simulink model "test_loopback_buf"  (Simulink 6.2)
settings: Solver=ode45  StartTime=0.0  StopTime=4000  RelTol=1e-3
undefined symbols (not defined in the file): Down, Up
libraries: xbsIndex_r3 x1383, xps_library x52, casper_library x37
(part 3 of 8)

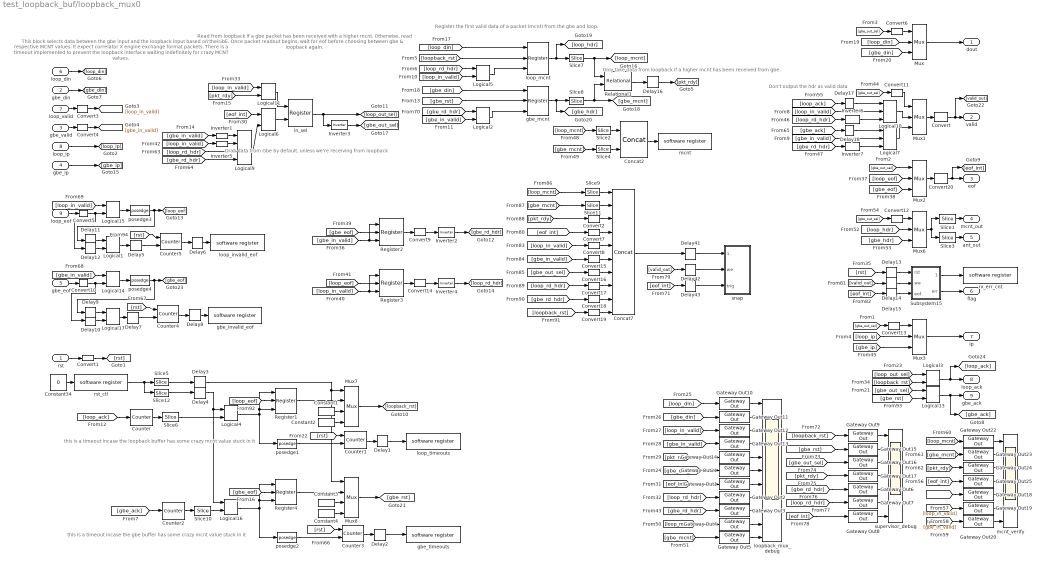
== system test_loopback_buf/loopback_mux0 ==
  note: Read from loopback if a gbe packet
      | has been received with a higher mcnt.
      | Otherwise, read from GbE.
      | Once packet readout begins, wait for eof
      | before choosing between gbe & loopback again.
  note: Only take data from loopback
      | if a higher mcnt has been
      | received from gbe.
  note: This block selects data between the gbe input
      | and the loopback input based on their respective MCNT values.
      | It expect correlator X engine exchange format packets.
      |
      | There is a timeout implemented to prevent the loopback interface
      | waiting indefinitely for crazy MCNT values.
  note: Don't output the hdr
      | as valid data
  note: this is a timeout incase
      | the gbe buffer has
      | some crazy mcnt value stuck in it
  note: this is a timeout incase
      | the loopback buffer has
      | some crazy mcnt value stuck in it
  note: Grab data from
      | Gbe by default,
      | unless we're receiving
      | from loopback
  note: Register the first valid
      | data of a packet (mcnt)
      | from the gbe and loop.
  rst : Inport  Port=1  LatchInput=off
  gbe_din : Inport  Port=2  LatchInput=off
  gbe_valid : Inport  Port=3  LatchInput=off
  gbe_ip : Inport  Port=4  LatchInput=off
  gbe_eof : Inport  Port=5  LatchInput=off
  loop_din : Inport  Port=6  LatchInput=off
  loop_valid : Inport  Port=7  LatchInput=off
  loop_ip : Inport  Port=8  LatchInput=off
  loop_eof : Inport  Port=9  LatchInput=off
  Concat2 : xbsIndex_r3/Concat  num_inputs=2  explicit_period=off  period=1  dbl_ovrd=off
  Concat7 : xbsIndex_r3/Concat  num_inputs=10  explicit_period=off  period=1  dbl_ovrd=off
  Constant1 : xbsIndex_r3/Constant  const=0  equ=P=C  arith_type=Boolean  n_bits=1  bin_pt=0  opselect=C  inp2=PCIN>>17  opr=+  inp1=P  carry=CIN  iostate=0  explicit_period=on  period=1  dbl_ovrd=off
  Constant2 : xbsIndex_r3/Constant  const=1  equ=P=C  arith_type=Boolean  n_bits=1  bin_pt=0  opselect=C  inp2=PCIN>>17  opr=+  inp1=P  carry=CIN  iostate=0  explicit_period=on  period=1  dbl_ovrd=off
  Constant3 : xbsIndex_r3/Constant  const=0  equ=P=C  arith_type=Boolean  n_bits=1  bin_pt=0  opselect=C  inp2=PCIN>>17  opr=+  inp1=P  carry=CIN  iostate=0  explicit_period=on  period=1  dbl_ovrd=off
  Constant34 : Constant  Value=0
  Constant4 : xbsIndex_r3/Constant  const=1  equ=P=C  arith_type=Boolean  n_bits=1  bin_pt=0  opselect=C  inp2=PCIN>>17  opr=+  inp1=P  carry=CIN  iostate=0  explicit_period=on  period=1  dbl_ovrd=off
  Convert{,1,9,14,20} (5 alike) : xbsIndex_r3/Convert  arith_type=Boolean  n_bits=8  bin_pt=6  quantization=Truncate  overflow=Wrap  latency=0  explicit_period=off  period=1  dbl_ovrd=off  show_param=off  inserted_by_tool=off  pipeline=off
      settings: xl_area=[0, 0, 0, 0, 0, 0, 0]
  Convert{3..5,10} (4 alike) : xbsIndex_r3/Convert  arith_type=Boolean  n_bits=1  bin_pt=0  quantization=Truncate  overflow=Wrap  latency=0  explicit_period=on  period=1  dbl_ovrd=off  show_param=off  inserted_by_tool=off  pipeline=off
      settings: xl_area=[0, 0, 0, 0, 0, 0, 0]
  Convert{2,6..8,11..13,15..19} (12 alike) : xbsIndex_r3/Convert  arith_type=Unsigned  n_bits=1  bin_pt=0  quantization=Truncate  overflow=Wrap  latency=0  explicit_period=off  period=1  dbl_ovrd=off  show_param=off  inserted_by_tool=off  pipeline=off
      settings: xl_area=[0, 0, 0, 0, 0, 0, 0]
  Counter : xbsIndex_r3/Counter  cnt_type=Free Running  n_bits=timeout_bits+1  bin_pt=0  arith_type=Unsigned  start_count=0  cnt_to=Inf  cnt_by_val=1  operation=Up  explicit_period=off  period=1  load_pin=off  rst=on  en=off  dbl_ovrd=off  show_param=off  use_rpm=on  gen_core=off
      settings: xl_area=[0, 0, 0, 0, 0, 0, 0]
  Counter{1,3..5} (4 alike) : xbsIndex_r3/Counter  cnt_type=Free Running  n_bits=27  bin_pt=0  arith_type=Unsigned  start_count=0  cnt_to=Inf  cnt_by_val=1  operation=Up  explicit_period=off  period=1  load_pin=off  rst=on  en=on  dbl_ovrd=off  show_param=off  use_rpm=on  gen_core=off
      settings: xl_area=[0, 0, 0, 0, 0, 0, 0]
  Counter2 : xbsIndex_r3/Counter  cnt_type=Free Running  n_bits=timeout_bits+1  bin_pt=0  arith_type=Unsigned  start_count=0  cnt_to=Inf  cnt_by_val=1  operation=Up  explicit_period=off  period=1  load_pin=off  rst=on  en=off  dbl_ovrd=off  show_param=off  use_rpm=on  gen_core=off
      settings: xl_area=[0, 0, 0, 0, 0, 0, 0]
  Delay{1..15} (15 alike) : xbsIndex_r3/Delay  latency=2  reg_retiming=on  explicit_period=on  period=1  en=off  accept_only_valid=off  init_zero=on  dbl_ovrd=off  show_param=off
      settings: xl_area=[0, 0, 0, 0, 0, 0, 0]
  Delay16 : xbsIndex_r3/Delay  latency=1  reg_retiming=on  explicit_period=on  period=1  en=off  accept_only_valid=off  init_zero=on  dbl_ovrd=off  show_param=off
      settings: xl_area=[0, 0, 0, 0, 0, 0, 0]
  Delay17 : xbsIndex_r3/Delay  latency=1  reg_retiming=on  explicit_period=on  period=1  en=off  accept_only_valid=off  init_zero=on  dbl_ovrd=off  show_param=off
      settings: xl_area=[0, 0, 0, 0, 0, 0, 0]
  Delay18 : xbsIndex_r3/Delay  latency=1  reg_retiming=on  explicit_period=on  period=1  en=off  accept_only_valid=off  init_zero=on  dbl_ovrd=off  show_param=off
      settings: xl_area=[0, 0, 0, 0, 0, 0, 0]
  Delay41 : xbsIndex_r3/Delay  latency=3  reg_retiming=on  explicit_period=on  period=1  en=off  accept_only_valid=off  init_zero=on  dbl_ovrd=off  show_param=off
      settings: xl_area=[0, 0, 0, 0, 0, 0, 0]
  Delay42 : xbsIndex_r3/Delay  latency=3  reg_retiming=on  explicit_period=on  period=1  en=off  accept_only_valid=off  init_zero=on  dbl_ovrd=off  show_param=off
      settings: xl_area=[0, 0, 0, 0, 0, 0, 0]
  Delay43 : xbsIndex_r3/Delay  latency=3  reg_retiming=on  explicit_period=on  period=1  en=off  accept_only_valid=off  init_zero=on  dbl_ovrd=off  show_param=off
      settings: xl_area=[0, 0, 0, 0, 0, 0, 0]
  Gateway Out{1..25} (25 alike) : xbsIndex_r3/Gateway Out  output_type=Double  nbits=8  bin_pt=6  arith_type=Boolean  quantization=Truncate  overflow=Wrap  hdl_port=on  timing_constraint=None  locs_specified=off  LOCs={}  needs_fixed_name=off  show_param=off
      settings: xl_area=[0, 0, 0, 0, 0, 0, 0]
  Inverter{1..7} (7 alike) : xbsIndex_r3/Inverter  latency=0  explicit_period=off  period=1  en=off  dbl_ovrd=off  show_param=off
      settings: xl_area=[0, 0, 0, 0, 0, 0, 0]
  Logical1 : xbsIndex_r3/Logical  logical_function=XOR  inputs=2  precision=Full  arith_type=Unsigned  n_bits=8  bin_pt=2  align_bp=on  latency=0  explicit_period=on  period=1  en=off  dbl_ovrd=off  show_param=off
      settings: xl_area=[0, 0, 0, 0, 0, 0, 0]
  Logical10 : xbsIndex_r3/Logical  logical_function=AND  inputs=3  precision=Full  arith_type=Unsigned  n_bits=8  bin_pt=2  align_bp=on  latency=0  explicit_period=on  period=1  en=off  dbl_ovrd=off  show_param=off
      settings: xl_area=[0, 0, 0, 0, 0, 0, 0]
  Logical11 : xbsIndex_r3/Logical  logical_function=AND  inputs=2  precision=Full  arith_type=Unsigned  n_bits=8  bin_pt=2  align_bp=on  latency=0  explicit_period=off  period=1  en=off  dbl_ovrd=off  show_param=off
      settings: xl_area=[0, 0, 0, 0, 0, 0, 0]
  Logical13 : xbsIndex_r3/Logical  logical_function=OR  inputs=2  precision=Full  arith_type=Unsigned  n_bits=8  bin_pt=2  align_bp=on  latency=0  explicit_period=off  period=1  en=off  dbl_ovrd=off  show_param=off
      settings: xl_area=[0, 0, 0, 0, 0, 0, 0]
  Logical14 : xbsIndex_r3/Logical  logical_function=AND  inputs=2  precision=Full  arith_type=Unsigned  n_bits=8  bin_pt=2  align_bp=on  latency=0  explicit_period=on  period=1  en=off  dbl_ovrd=off  show_param=off
      settings: xl_area=[0, 0, 0, 0, 0, 0, 0]
  Logical15 : xbsIndex_r3/Logical  logical_function=AND  inputs=2  precision=Full  arith_type=Unsigned  n_bits=8  bin_pt=2  align_bp=on  latency=0  explicit_period=on  period=1  en=off  dbl_ovrd=off  show_param=off
      settings: xl_area=[0, 0, 0, 0, 0, 0, 0]
  Logical16 : xbsIndex_r3/Logical  logical_function=OR  inputs=2  precision=Full  arith_type=Unsigned  n_bits=8  bin_pt=2  align_bp=on  latency=0  explicit_period=on  period=1  en=off  dbl_ovrd=off  show_param=off
      settings: xl_area=[0, 0, 0, 0, 0, 0, 0]
  Logical17 : xbsIndex_r3/Logical  logical_function=XOR  inputs=2  precision=Full  arith_type=Unsigned  n_bits=8  bin_pt=2  align_bp=on  latency=0  explicit_period=on  period=1  en=off  dbl_ovrd=off  show_param=off
      settings: xl_area=[0, 0, 0, 0, 0, 0, 0]
  Logical2 : xbsIndex_r3/Logical  logical_function=AND  inputs=2  precision=Full  arith_type=Unsigned  n_bits=8  bin_pt=2  align_bp=on  latency=0  explicit_period=off  period=1  en=off  dbl_ovrd=off  show_param=off
      settings: xl_area=[0, 0, 0, 0, 0, 0, 0]
  Logical3 : xbsIndex_r3/Logical  logical_function=OR  inputs=2  precision=Full  arith_type=Unsigned  n_bits=8  bin_pt=2  align_bp=on  latency=0  explicit_period=off  period=1  en=off  dbl_ovrd=off  show_param=off
      settings: xl_area=[0, 0, 0, 0, 0, 0, 0]
  Logical4 : xbsIndex_r3/Logical  logical_function=OR  inputs=2  precision=Full  arith_type=Unsigned  n_bits=8  bin_pt=2  align_bp=on  latency=0  explicit_period=on  period=1  en=off  dbl_ovrd=off  show_param=off
      settings: xl_area=[0, 0, 0, 0, 0, 0, 0]
  Logical5 : xbsIndex_r3/Logical  logical_function=AND  inputs=2  precision=Full  arith_type=Unsigned  n_bits=8  bin_pt=2  align_bp=on  latency=0  explicit_period=off  period=1  en=off  dbl_ovrd=off  show_param=off
      settings: xl_area=[0, 0, 0, 0, 0, 0, 0]
  Logical6 : xbsIndex_r3/Logical  logical_function=OR  inputs=2  precision=Full  arith_type=Unsigned  n_bits=8  bin_pt=2  align_bp=on  latency=0  explicit_period=off  period=1  en=off  dbl_ovrd=off  show_param=off
      settings: xl_area=[0, 0, 0, 0, 0, 0, 0]
  Logical7 : xbsIndex_r3/Logical  logical_function=AND  inputs=3  precision=Full  arith_type=Unsigned  n_bits=8  bin_pt=2  align_bp=on  latency=0  explicit_period=on  period=1  en=off  dbl_ovrd=off  show_param=off
      settings: xl_area=[0, 0, 0, 0, 0, 0, 0]
  Logical9 : xbsIndex_r3/Logical  logical_function=AND  inputs=4  precision=Full  arith_type=Unsigned  n_bits=8  bin_pt=2  align_bp=on  latency=0  explicit_period=on  period=1  en=off  dbl_ovrd=off  show_param=off
      settings: xl_area=[0, 0, 0, 0, 0, 0, 0]
  Mux{,1,3,6} (4 alike) : xbsIndex_r3/Mux  inputs=2  precision=Full  arith_type="Signed  (2's comp)"  n_bits=8  bin_pt=2  quantization=Truncate  overflow=Wrap  latency=0  explicit_period=off  period=1  en=off  dbl_ovrd=off  show_param=off  mux_type=off  use_rpm=off  gen_core=off
      settings: xl_area=[0, 0, 0, 0, 0, 0, 0]
  Mux2 : xbsIndex_r3/Mux  inputs=2  precision=Full  arith_type="Signed  (2's comp)"  n_bits=8  bin_pt=2  quantization=Truncate  overflow=Wrap  latency=0  explicit_period=on  period=1  en=off  dbl_ovrd=off  show_param=off  mux_type=off  use_rpm=off  gen_core=off
      settings: xl_area=[0, 0, 0, 0, 0, 0, 0]
  Mux7 : xbsIndex_r3/Mux  inputs=3  precision=Full  arith_type="Signed  (2's comp)"  n_bits=8  bin_pt=2  quantization=Truncate  overflow=Wrap  latency=2  explicit_period=off  period=1  en=off  dbl_ovrd=off  show_param=off  mux_type=off  use_rpm=off  gen_core=off
      settings: xl_area=[0, 0, 0, 0, 0, 0, 0]
  Mux8 : xbsIndex_r3/Mux  inputs=3  precision=Full  arith_type="Signed  (2's comp)"  n_bits=8  bin_pt=2  quantization=Truncate  overflow=Wrap  latency=2  explicit_period=off  period=1  en=off  dbl_ovrd=off  show_param=off  mux_type=off  use_rpm=off  gen_core=off
      settings: xl_area=[0, 0, 0, 0, 0, 0, 0]
  Register{1..4} (4 alike) : xbsIndex_r3/Register  init=0  reg_only_valid=off  explicit_period=on  period=1  rst=on  en=on  out_en=off  dbl_ovrd=off  show_param=off
      settings: xl_area=[0, 0, 0, 0, 0, 0, 0]
  Relational1 : xbsIndex_r3/Relational  mode=a<b  latency=1  explicit_period=off  period=1  en=off  dbl_ovrd=off  show_param=off
      settings: xl_area=[0, 0, 0, 0, 0, 0, 0]
  Slice1 : xbsIndex_r3/Slice  mode=Lower Bit Location + Width  nbits=48  bit1=0  base1=MSB of Input  bit0=16  base0=LSB of Input  boolean_output=off  explicit_period=off  period=1  dbl_ovrd=off
  Slice10 : xbsIndex_r3/Slice  mode=Upper Bit Location + Width  nbits=1  bit1=0  base1=MSB of Input  bit0=1  base0=LSB of Input  boolean_output=on  explicit_period=off  period=1  dbl_ovrd=off
  Slice11 : xbsIndex_r3/Slice  mode=Lower Bit Location + Width  nbits=12  bit1=0  base1=MSB of Input  bit0=0  base0=LSB of Input  boolean_output=off  explicit_period=off  period=1  dbl_ovrd=off
  Slice12 : xbsIndex_r3/Slice  mode=Lower Bit Location + Width  nbits=1  bit1=0  base1=MSB of Input  bit0=0  base0=LSB of Input  boolean_output=on  explicit_period=off  period=1  dbl_ovrd=off
  Slice2 : xbsIndex_r3/Slice  mode=Lower Bit Location + Width  nbits=16  bit1=0  base1=MSB of Input  bit0=0  base0=LSB of Input  boolean_output=off  explicit_period=off  period=1  dbl_ovrd=off
  Slice3 : xbsIndex_r3/Slice  mode=Lower Bit Location + Width  nbits=16  bit1=0  base1=MSB of Input  bit0=0  base0=LSB of Input  boolean_output=off  explicit_period=off  period=1  dbl_ovrd=off
  Slice4 : xbsIndex_r3/Slice  mode=Lower Bit Location + Width  nbits=16  bit1=0  base1=MSB of Input  bit0=0  base0=LSB of Input  boolean_output=off  explicit_period=off  period=1  dbl_ovrd=off
  Slice5 : xbsIndex_r3/Slice  mode=Lower Bit Location + Width  nbits=2  bit1=0  base1=MSB of Input  bit0=1  base0=LSB of Input  boolean_output=off  explicit_period=off  period=1  dbl_ovrd=off
  Slice6 : xbsIndex_r3/Slice  mode=Upper Bit Location + Width  nbits=1  bit1=0  base1=MSB of Input  bit0=1  base0=LSB of Input  boolean_output=on  explicit_period=off  period=1  dbl_ovrd=off
  Slice7 : xbsIndex_r3/Slice  mode=Upper Bit Location + Width  nbits=48  bit1=0  base1=MSB of Input  bit0=0  base0=LSB of Input  boolean_output=off  explicit_period=off  period=1  dbl_ovrd=off
  Slice8 : xbsIndex_r3/Slice  mode=Upper Bit Location + Width  nbits=48  bit1=0  base1=MSB of Input  bit0=0  base0=LSB of Input  boolean_output=off  explicit_period=off  period=1  dbl_ovrd=off
  Slice9 : xbsIndex_r3/Slice  mode=Lower Bit Location + Width  nbits=12  bit1=0  base1=MSB of Input  bit0=0  base0=LSB of Input  boolean_output=off  explicit_period=off  period=1  dbl_ovrd=off
  Subsystem15 : Subsystem  mask{payload_len=payload_len}
      mask init:
      | fmtstr = sprintf('Payload Length: %d', payload_len);
      | set_param(gcb, 'AttributesFormatString', fmtstr);
      settings: AttributesFormatString=Payload Length: 32
  gbe_invalid_eof : xps_library/software register  Tag=xps:sw_reg  io_dir=To Processor  arith_type=Unsigned  bitwidth=32  bin_pt=0  sample_period=1  gw_name=b_2x_8a_r310_a_loopback_mux0_gbe_invalid_eof_user_data_in
  gbe_mcnt : xbsIndex_r3/Register  init=0  reg_only_valid=off  explicit_period=on  period=1  rst=on  en=on  out_en=off  dbl_ovrd=off  show_param=off
      settings: xl_area=[0, 0, 0, 0, 0, 0, 0]
  gbe_timeouts : xps_library/software register  Tag=xps:sw_reg  io_dir=To Processor  arith_type=Unsigned  bitwidth=32  bin_pt=0  sample_period=1  gw_name=b_2x_8a_r310_a_loopback_mux0_gbe_timeouts_user_data_in
  in_sel : xbsIndex_r3/Register  init=0  reg_only_valid=off  explicit_period=on  period=1  rst=off  en=on  out_en=off  dbl_ovrd=off  show_param=off
      settings: xl_area=[0, 0, 0, 0, 0, 0, 0]
  loop_invalid_eof : xps_library/software register  Tag=xps:sw_reg  io_dir=To Processor  arith_type=Unsigned  bitwidth=32  bin_pt=0  sample_period=1  gw_name=b_2x_8a_r310_a_loopback_mux0_loop_invalid_eof_user_data_in
  loop_mcnt : xbsIndex_r3/Register  init=0  reg_only_valid=off  explicit_period=on  period=1  rst=on  en=on  out_en=off  dbl_ovrd=off  show_param=off
      settings: xl_area=[0, 0, 0, 0, 0, 0, 0]
  loop_timeouts : xps_library/software register  Tag=xps:sw_reg  io_dir=To Processor  arith_type=Unsigned  bitwidth=32  bin_pt=0  sample_period=1  gw_name=b_2x_8a_r310_a_loopback_mux0_loop_timeouts_user_data_in
  loopback_mux_debug : Scope  NumInputPorts=11
      settings: YMin=300~190.95~0~0.95~0.95~-1~-1~-1~-5~-5~-5  YMax=525~211.05~1~1.05~1.05~1~1~1~5~5~5  SaveName=ScopeData7
  mcnt : xps_library/software register  Tag=xps:sw_reg  io_dir=To Processor  arith_type=Unsigned  bitwidth=32  bin_pt=0  sample_period=1  gw_name=b_2x_8a_r310_a_loopback_mux0_mcnt_user_data_in
  mcnt_verify : Scope  NumInputPorts=7
      settings: YMin=300~190.95~0~-5~-5~-5~-5  YMax=525~211.05~1~5~5~5~5  SaveName=ScopeData2
  posedge{1..4} (4 alike) : casper_library/Misc/posedge  Tag=Rising Edge Detector
  rst_ctl : xps_library/software register  Tag=xps:sw_reg  io_dir=From Processor  arith_type=Unsigned  bitwidth=32  bin_pt=0  sample_period=1  gw_name=b_2x_8a_r310_a_loopback_mux0_rst_ctl_user_data_out
  rx_err_cnt : xps_library/software register  Tag=xps:sw_reg  io_dir=To Processor  arith_type=Unsigned  bitwidth=32  bin_pt=0  sample_period=1  gw_name=b_2x_8a_r310_a_loopback_mux0_rx_err_cnt_user_data_in
  snap : Subsystem  mask{nsamples=12}
      mask prompts: nsamples "Number of Samples (2^?)"
  supervisor_debug : Scope  NumInputPorts=7
      settings: YMin=300~190.95~0~-5~-5~-5~-5  YMax=525~211.05~1~5~5~5~5  SaveName=ScopeData18
  dout : Outport
  valid : Outport  Port=2
  eof : Outport  Port=3
  mcnt_out : Outport  Port=4
  ant_out : Outport  Port=5
  flag : Outport  Port=6
  ip : Outport  Port=7
  loop_ack : Outport  Port=8
  gbe_ack : Outport  Port=9
  wires:
  Mux/1 -> dout/1
  Mux1/1 -> Convert/1
  Mux2/1 -> Convert20/1
  gbe_valid/1 -> Convert4/1
  loop_valid/1 -> Convert3/1
  Convert/1 -> valid/1, [valid_out]
  Slice2/1 -> Concat2/1
  Slice4/1 -> Concat2/2
  Concat2/1 -> mcnt/1
  Convert6/1 -> Mux/1
  [gbe_out_sel] -> Convert6/1
  [gbe_out_sel] -> Mux2/1
  Gateway Out12/1 -> loopback_mux_debug/3
  Gateway Out13/1 -> loopback_mux_debug/4
  Gateway Out14/1 -> loopback_mux_debug/5
  Gateway Out21/1 -> loopback_mux_debug/6
  Convert3/1 -> [loop_in_valid]
  Convert4/1 -> [gbe_in_valid]
  Relational1/1 -> Delay16/1
  loop_din/1 -> [loop_din]
  gbe_din/1 -> [gbe_din]
  [loop_din] -> Mux/2
  [gbe_din] -> Mux/3
  [gbe_din] -> Gateway Out11/1
  [loop_din] -> Gateway Out10/1
  [loop_in_valid] -> Gateway Out12/1
  [gbe_in_valid] -> Gateway Out13/1
  [gbe_out_sel] -> Gateway Out21/1
  [pkt_rdy] -> Gateway Out14/1
  Gateway Out1/1 -> loopback_mux_debug/7
  [eof_int] -> Gateway Out1/1
  [loop_rd_hdr] -> Gateway Out2/1
  Gateway Out2/1 -> loopback_mux_debug/8
  [loop_eof] -> Mux2/2
  loop_eof/1 -> Convert5/1
  gbe_eof/1 -> Convert10/1
  [gbe_eof] -> Mux2/3
  Gateway Out3/1 -> loopback_mux_debug/9
  [gbe_rd_hdr] -> Gateway Out3/1
  [gbe_out_sel] -> Convert11/1
  Convert11/1 -> Mux1/1
  loop_ip/1 -> [loop_ip]
  gbe_ip/1 -> [gbe_ip]
  Mux3/1 -> ip/1
  [loop_ip] -> Mux3/2
  [gbe_ip] -> Mux3/3
  [gbe_out_sel] -> Convert13/1
  Convert13/1 -> Mux3/1
  [loop_mcnt] -> Slice2/1
  [gbe_mcnt] -> Slice4/1
  Gateway Out10/1 -> loopback_mux_debug/1
  Gateway Out11/1 -> loopback_mux_debug/2
  Gateway Out4/1 -> loopback_mux_debug/10
  Gateway Out5/1 -> loopback_mux_debug/11
  [loop_mcnt] -> Gateway Out4/1
  [gbe_mcnt] -> Gateway Out5/1
  Gateway Out24/1 -> mcnt_verify/3
  Gateway Out22/1 -> mcnt_verify/1
  Gateway Out23/1 -> mcnt_verify/2
  Gateway Out25/1 -> mcnt_verify/4
  Gateway Out18/1 -> mcnt_verify/5
  Gateway Out19/1 -> mcnt_verify/6
  Gateway Out20/1 -> mcnt_verify/7
  [gbe_out_sel] -> Gateway Out20/1
  [gbe_in_valid] -> Gateway Out19/1
  [loop_in_valid] -> Gateway Out18/1
  [eof_int] -> Gateway Out25/1
  [loop_mcnt] -> Gateway Out22/1
  [gbe_mcnt] -> Gateway Out23/1
  [pkt_rdy] -> Gateway Out24/1
  Slice7/1 -> Relational1/1, [loop_mcnt]
  Slice8/1 -> Relational1/2, [gbe_mcnt]
  Slice1/1 -> mcnt_out/1
  Slice3/1 -> ant_out/1
  Convert12/1 -> Mux6/1
  [gbe_out_sel] -> Convert12/1
  [loop_hdr] -> Mux6/2
  [gbe_hdr] -> Mux6/3
  Mux6/1 -> Slice1/1, Slice3/1
  [loop_in_valid] -> Logical10/2
  [loop_ack] -> Delay17/1
  [gbe_ack] -> Delay18/1
  [gbe_in_valid] -> Logical7/2
  Logical7/1 -> Mux1/3
  Counter2/1 -> Slice10/1
  [gbe_ack] -> Counter2/1
  [rst] -> Counter3/1
  Counter3/1 -> Delay2/1
  Logical16/1 -> Register4/1, Register4/3, posedge2/1
  Logical14/1 -> posedge4/1
  Logical15/1 -> posedge3/1
  Convert5/1 -> Logical15/2, Delay12/1
  Convert10/1 -> Logical14/2, Delay10/1
  [gbe_in_valid] -> Logical14/1
  [loop_in_valid] -> Logical15/1
  Slice10/1 -> Logical16/2
  Gateway Out16/1 -> supervisor_debug/3
  Gateway Out9/1 -> supervisor_debug/1
  Gateway Out15/1 -> supervisor_debug/2
  Gateway Out17/1 -> supervisor_debug/4
  Gateway Out6/1 -> supervisor_debug/5
  Gateway Out7/1 -> supervisor_debug/6
  Gateway Out8/1 -> supervisor_debug/7
  [loopback_rst] -> Gateway Out9/1
  [gbe_rst] -> Gateway Out15/1
  [gbe_out_sel] -> Gateway Out16/1
  [pkt_rdy] -> Gateway Out17/1
  [gbe_rd_hdr] -> Gateway Out6/1
  [loop_rd_hdr] -> Gateway Out7/1
  [eof_int] -> Gateway Out8/1
  Logical3/1 -> loop_ack/1, [loop_ack]
  Logical13/1 -> gbe_ack/1, [gbe_ack]
  rst/1 -> Convert1/1
  Subsystem15/1(err_cnt) -> rx_err_cnt/1
  Subsystem15/2(err) -> flag/1
  [rst] -> Delay13/1
  [valid_out] -> Delay14/1
  [eof_int] -> Delay15/1
  Counter/1 -> Slice6/1
  Slice6/1 -> Logical4/2
  [loop_ack] -> Counter/1
  [rst] -> Counter1/1
  Counter1/1 -> Delay1/1
  Logical4/1 -> Register1/1, Register1/3, posedge1/1
  [pkt_rdy] -> Logical11/2
  [eof_int] -> Logical6/1
  Inverter3/1 -> [gbe_out_sel]
  in_sel/1 -> Inverter3/1, [loop_out_sel]
  Logical6/1 -> in_sel/2
  [loop_in_valid] -> Logical11/1
  Register2/1 -> Convert9/1
  Convert9/1 -> Inverter2/1
  Inverter2/1 -> [gbe_rd_hdr]
  [gbe_eof] -> Register2/2
  Register3/1 -> Convert14/1
  Convert14/1 -> Inverter4/1
  Inverter4/1 -> [loop_rd_hdr]
  [loop_eof] -> Register3/2
  Logical11/1 -> in_sel/1
  [gbe_in_valid] -> Register2/1, Register2/3
  [loop_in_valid] -> Register3/1, Register3/3
  [gbe_in_valid] -> Inverter1/1
  [loop_in_valid] -> Inverter5/1
  Logical9/1 -> Logical6/2
  Inverter1/1 -> Logical9/1
  Inverter5/1 -> Logical9/2
  [loop_rd_hdr] -> Logical9/3
  [gbe_rd_hdr] -> Logical9/4
  gbe_mcnt/1 -> Slice8/1, [gbe_hdr]
  loop_mcnt/1 -> Slice7/1, [loop_hdr]
  Logical5/1 -> loop_mcnt/3
  [loop_rd_hdr] -> Logical5/1
  [gbe_rd_hdr] -> Logical2/1
  [loop_in_valid] -> Logical5/2
  [gbe_in_valid] -> Logical2/2
  [loop_din] -> loop_mcnt/1
  [gbe_din] -> gbe_mcnt/1
  Concat7/1 -> Delay41/1
  Delay42/1 -> snap/2(we)
  Delay43/1 -> snap/3(trig)
  Delay41/1 -> snap/1(data_in)
  [valid_out] -> Delay42/1
  [eof_int] -> Delay43/1
  [loop_mcnt] -> Slice9/1
  [gbe_mcnt] -> Slice11/1
  Slice9/1 -> Concat7/1
  Slice11/1 -> Concat7/2
  [pkt_rdy] -> Convert2/1
  [eof_int] -> Convert7/1
  [loop_in_valid] -> Convert8/1
  [gbe_in_valid] -> Convert15/1
  [gbe_out_sel] -> Convert16/1
  [loop_rd_hdr] -> Convert17/1
  [gbe_rd_hdr] -> Convert18/1
  [loopback_rst] -> Convert19/1
  [loop_eof] -> Register1/2
  [gbe_eof] -> Register4/2
  [loop_out_sel] -> Logical3/1
  [gbe_out_sel] -> Logical13/1
  [loopback_rst] -> Logical3/2
  [gbe_rst] -> Logical13/2
  Mux7/1 -> [loopback_rst]
  Register1/1 -> Mux7/2
  Mux8/1 -> [gbe_rst]
  Register4/1 -> Mux8/2
  Constant1/1 -> Mux7/3
  Constant34/1 -> rst_ctl/1
  rst_ctl/1 -> Slice5/1, Slice12/1
  Slice5/1 -> Delay3/1
  Convert1/1 -> [rst]
  Slice12/1 -> Delay4/1
  [loopback_rst] -> loop_mcnt/2
  [gbe_rst] -> gbe_mcnt/2
  Convert2/1 -> Concat7/3
  Convert7/1 -> Concat7/4
  Convert8/1 -> Concat7/5
  Convert15/1 -> Concat7/6
  Convert16/1 -> Concat7/7
  Convert17/1 -> Concat7/8
  Convert18/1 -> Concat7/9
  Convert19/1 -> Concat7/10
  Convert20/1 -> [eof_int], eof/1
  posedge1/1 -> Counter1/2
  posedge2/1 -> Counter3/2
  posedge3/1 -> [loop_eof], Delay11/1
  posedge4/1 -> [gbe_eof], Delay9/1
  [rst] -> Counter5/1
  Counter5/1 -> Delay6/1
  Logical1/1 -> Delay5/1
  Constant2/1 -> Mux7/4
  Constant3/1 -> Mux8/3
  Constant4/1 -> Mux8/4
  Delay1/1 -> loop_timeouts/1
  Delay2/1 -> gbe_timeouts/1
  Delay3/1 -> Mux7/1, Mux8/1
  Delay4/1 -> Logical4/1, Logical16/1
  Delay5/1 -> Counter5/2
  Delay6/1 -> loop_invalid_eof/1
  [rst] -> Counter4/1
  Counter4/1 -> Delay8/1
  Logical17/1 -> Delay7/1
  Delay7/1 -> Counter4/2
  Delay8/1 -> gbe_invalid_eof/1
  Delay9/1 -> Logical17/1
  Delay10/1 -> Logical17/2
  Delay11/1 -> Logical1/1
  Delay12/1 -> Logical1/2
  Delay13/1 -> Subsystem15/1(rst)
  Delay14/1 -> Subsystem15/2(we)
  Delay15/1 -> Subsystem15/3(eof)
  Logical2/1 -> gbe_mcnt/3
  Delay16/1 -> [pkt_rdy]
  Delay17/1 -> Logical10/1
  Delay18/1 -> Logical7/1
  Inverter6/1 -> Logical10/3
  [loop_rd_hdr] -> Inverter6/1
  [gbe_rd_hdr] -> Inverter7/1
  Inverter7/1 -> Logical7/3
  Logical10/1 -> Mux1/2

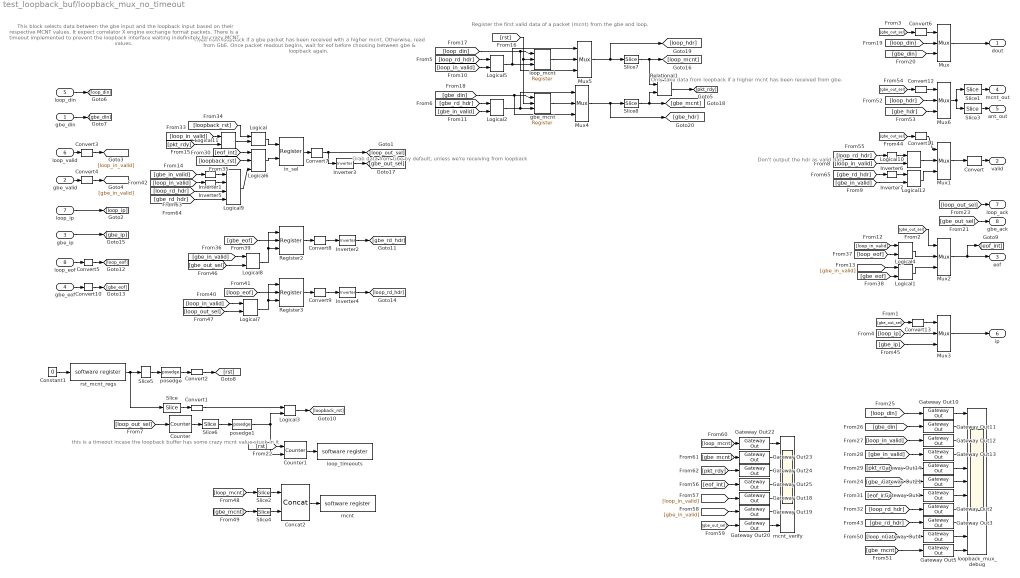
== system test_loopback_buf/loopback_mux_no_timeout ==
  note: Read from loopback if a gbe packet
      | has been received with a higher mcnt.
      | Otherwise, read from GbE.
      | Once packet readout begins, wait for eof
      | before choosing between gbe & loopback again.
  note: Register the first valid
      | data of a packet (mcnt)
      | from the gbe and loop.
  note: Only take data from loopback
      | if a higher mcnt has been
      | received from gbe.
  note: This block selects data between the gbe input
      | and the loopback input based on their respective MCNT values.
      | It expect correlator X engine exchange format packets.
      |
      | There is a timeout implemented to prevent the loopback interface
      | waiting indefinitely for crazy MCNT values.
  note: this is a timeout incase
      | the loopback buffer has
      | some crazy mcnt value stuck in it
  note: Grab data from
      | Gbe by default,
      | unless we're receiving
      | from loopback
  note: Don't output the hdr
      | as valid data
  gbe_din : Inport  Port=1  LatchInput=off
  gbe_valid : Inport  Port=2  LatchInput=off
  gbe_ip : Inport  Port=3  LatchInput=off
  gbe_eof : Inport  Port=4  LatchInput=off
  loop_din : Inport  Port=5  LatchInput=off
  loop_valid : Inport  Port=6  LatchInput=off
  loop_ip : Inport  Port=7  LatchInput=off
  loop_eof : Inport  Port=8  LatchInput=off
  Concat2 : xbsIndex_r3/Concat  num_inputs=2  explicit_period=off  period=1  dbl_ovrd=off
  Constant1 : Constant  Value=0
  Convert{,1..2,7..9} (6 alike) : xbsIndex_r3/Convert  arith_type=Boolean  n_bits=8  bin_pt=6  quantization=Truncate  overflow=Wrap  latency=0  explicit_period=off  period=1  dbl_ovrd=off  show_param=off  inserted_by_tool=off  pipeline=off
      settings: xl_area=[0, 0, 0, 0, 0, 0, 0]
  Convert{3..5,10} (4 alike) : xbsIndex_r3/Convert  arith_type=Boolean  n_bits=1  bin_pt=0  quantization=Truncate  overflow=Wrap  latency=0  explicit_period=on  period=1  dbl_ovrd=off  show_param=off  inserted_by_tool=off  pipeline=off
      settings: xl_area=[0, 0, 0, 0, 0, 0, 0]
  Convert{6,11..13} (4 alike) : xbsIndex_r3/Convert  arith_type=Unsigned  n_bits=1  bin_pt=0  quantization=Truncate  overflow=Wrap  latency=0  explicit_period=off  period=1  dbl_ovrd=off  show_param=off  inserted_by_tool=off  pipeline=off
      settings: xl_area=[0, 0, 0, 0, 0, 0, 0]
  Counter : xbsIndex_r3/Counter  cnt_type=Free Running  n_bits=loopback_timeout + 1  bin_pt=0  arith_type=Unsigned  start_count=0  cnt_to=Inf  cnt_by_val=1  operation=Up  explicit_period=off  period=1  load_pin=off  rst=on  en=off  dbl_ovrd=off  show_param=off  use_rpm=on  gen_core=off
      settings: xl_area=[0, 0, 0, 0, 0, 0, 0]
  Counter1 : xbsIndex_r3/Counter  cnt_type=Free Running  n_bits=27  bin_pt=0  arith_type=Unsigned  start_count=0  cnt_to=Inf  cnt_by_val=1  operation=Up  explicit_period=off  period=1  load_pin=off  rst=on  en=on  dbl_ovrd=off  show_param=off  use_rpm=on  gen_core=off
      settings: xl_area=[0, 0, 0, 0, 0, 0, 0]
  Gateway Out{1..5,10..14,18..25} (18 alike) : xbsIndex_r3/Gateway Out  output_type=Double  nbits=8  bin_pt=6  arith_type=Boolean  quantization=Truncate  overflow=Wrap  hdl_port=on  timing_constraint=None  locs_specified=off  LOCs={}  needs_fixed_name=off  show_param=off
      settings: xl_area=[0, 0, 0, 0, 0, 0, 0]
  Inverter{1..7} (7 alike) : xbsIndex_r3/Inverter  latency=0  explicit_period=off  period=1  en=off  dbl_ovrd=off  show_param=off
      settings: xl_area=[0, 0, 0, 0, 0, 0, 0]
  Logical : xbsIndex_r3/Logical  logical_function=OR  inputs=2  precision=Full  arith_type=Unsigned  n_bits=8  bin_pt=2  align_bp=on  latency=0  explicit_period=off  period=1  en=off  dbl_ovrd=off  show_param=off
      settings: xl_area=[0, 0, 0, 0, 0, 0, 0]
  Logical{1,4,7..8,10} (5 alike) : xbsIndex_r3/Logical  logical_function=AND  inputs=2  precision=Full  arith_type=Unsigned  n_bits=8  bin_pt=2  align_bp=on  latency=0  explicit_period=on  period=1  en=off  dbl_ovrd=off  show_param=off
      settings: xl_area=[0, 0, 0, 0, 0, 0, 0]
  Logical{2,5,11..12} (4 alike) : xbsIndex_r3/Logical  logical_function=AND  inputs=2  precision=Full  arith_type=Unsigned  n_bits=8  bin_pt=2  align_bp=on  latency=0  explicit_period=off  period=1  en=off  dbl_ovrd=off  show_param=off
      settings: xl_area=[0, 0, 0, 0, 0, 0, 0]
  Logical3 : xbsIndex_r3/Logical  logical_function=OR  inputs=2  precision=Full  arith_type=Unsigned  n_bits=8  bin_pt=2  align_bp=on  latency=0  explicit_period=off  period=1  en=off  dbl_ovrd=off  show_param=off
      settings: xl_area=[0, 0, 0, 0, 0, 0, 0]
  Logical6 : xbsIndex_r3/Logical  logical_function=OR  inputs=3  precision=Full  arith_type=Unsigned  n_bits=8  bin_pt=2  align_bp=on  latency=0  explicit_period=off  period=1  en=off  dbl_ovrd=off  show_param=off
      settings: xl_area=[0, 0, 0, 0, 0, 0, 0]
  Logical9 : xbsIndex_r3/Logical  logical_function=AND  inputs=4  precision=Full  arith_type=Unsigned  n_bits=8  bin_pt=2  align_bp=on  latency=0  explicit_period=on  period=1  en=off  dbl_ovrd=off  show_param=off
      settings: xl_area=[0, 0, 0, 0, 0, 0, 0]
  Mux{,1,3..6} (6 alike) : xbsIndex_r3/Mux  inputs=2  precision=Full  arith_type="Signed  (2's comp)"  n_bits=8  bin_pt=2  quantization=Truncate  overflow=Wrap  latency=0  explicit_period=off  period=1  en=off  dbl_ovrd=off  show_param=off  mux_type=off  use_rpm=off  gen_core=off
      settings: xl_area=[0, 0, 0, 0, 0, 0, 0]
  Mux2 : xbsIndex_r3/Mux  inputs=2  precision=Full  arith_type="Signed  (2's comp)"  n_bits=8  bin_pt=2  quantization=Truncate  overflow=Wrap  latency=0  explicit_period=on  period=1  en=off  dbl_ovrd=off  show_param=off  mux_type=off  use_rpm=off  gen_core=off
      settings: xl_area=[0, 0, 0, 0, 0, 0, 0]
  Register2 : xbsIndex_r3/Register  init=0  reg_only_valid=off  explicit_period=on  period=1  rst=on  en=on  out_en=off  dbl_ovrd=off  show_param=off
      settings: xl_area=[0, 0, 0, 0, 0, 0, 0]
  Register3 : xbsIndex_r3/Register  init=0  reg_only_valid=off  explicit_period=on  period=1  rst=on  en=on  out_en=off  dbl_ovrd=off  show_param=off
      settings: xl_area=[0, 0, 0, 0, 0, 0, 0]
  Relational1 : xbsIndex_r3/Relational  mode=a<b  latency=0  explicit_period=off  period=1  en=off  dbl_ovrd=off  show_param=off
      settings: xl_area=[0, 0, 0, 0, 0, 0, 0]
  Slice : xbsIndex_r3/Slice  mode=Lower Bit Location + Width  nbits=1  bit1=0  base1=MSB of Input  bit0=1  base0=LSB of Input  boolean_output=off  explicit_period=off  period=1  dbl_ovrd=off
  Slice1 : xbsIndex_r3/Slice  mode=Lower Bit Location + Width  nbits=48  bit1=0  base1=MSB of Input  bit0=16  base0=LSB of Input  boolean_output=off  explicit_period=off  period=1  dbl_ovrd=off
  Slice2 : xbsIndex_r3/Slice  mode=Lower Bit Location + Width  nbits=16  bit1=0  base1=MSB of Input  bit0=0  base0=LSB of Input  boolean_output=off  explicit_period=off  period=1  dbl_ovrd=off
  Slice3 : xbsIndex_r3/Slice  mode=Lower Bit Location + Width  nbits=16  bit1=0  base1=MSB of Input  bit0=0  base0=LSB of Input  boolean_output=off  explicit_period=off  period=1  dbl_ovrd=off
  Slice4 : xbsIndex_r3/Slice  mode=Lower Bit Location + Width  nbits=16  bit1=0  base1=MSB of Input  bit0=0  base0=LSB of Input  boolean_output=off  explicit_period=off  period=1  dbl_ovrd=off
  Slice5 : xbsIndex_r3/Slice  mode=Lower Bit Location + Width  nbits=1  bit1=0  base1=MSB of Input  bit0=0  base0=LSB of Input  boolean_output=off  explicit_period=off  period=1  dbl_ovrd=off
  Slice6 : xbsIndex_r3/Slice  mode=Upper Bit Location + Width  nbits=1  bit1=0  base1=MSB of Input  bit0=1  base0=LSB of Input  boolean_output=on  explicit_period=off  period=1  dbl_ovrd=off
  Slice7 : xbsIndex_r3/Slice  mode=Upper Bit Location + Width  nbits=48  bit1=0  base1=MSB of Input  bit0=0  base0=LSB of Input  boolean_output=off  explicit_period=off  period=1  dbl_ovrd=off
  Slice8 : xbsIndex_r3/Slice  mode=Upper Bit Location + Width  nbits=48  bit1=0  base1=MSB of Input  bit0=0  base0=LSB of Input  boolean_output=off  explicit_period=off  period=1  dbl_ovrd=off
  gbe_mcnt : xbsIndex_r3/Register  init=0  reg_only_valid=off  explicit_period=on  period=1  rst=on  en=on  out_en=off  dbl_ovrd=off  show_param=off
      settings: xl_area=[0, 0, 0, 0, 0, 0, 0]
  in_sel : xbsIndex_r3/Register  init=0  reg_only_valid=off  explicit_period=on  period=1  rst=off  en=on  out_en=off  dbl_ovrd=off  show_param=off
      settings: xl_area=[0, 0, 0, 0, 0, 0, 0]
  loop_mcnt : xbsIndex_r3/Register  init=0  reg_only_valid=off  explicit_period=on  period=1  rst=on  en=on  out_en=off  dbl_ovrd=off  show_param=off
      settings: xl_area=[0, 0, 0, 0, 0, 0, 0]
  loop_timeouts : xps_library/software register  Tag=xps:sw_reg  io_dir=To Processor  arith_type=Unsigned  bitwidth=32  bin_pt=0  sample_period=1  gw_name=test_loopback_buf_loopback_mux_no_timeout_loop_timeouts_user_data_in
  loopback_mux_debug : Scope  NumInputPorts=11
      settings: YMin=300~190.95~0~0.95~0.95~-1~-1~-1~-5~-5~-5  YMax=525~211.05~1~1.05~1.05~1~1~1~5~5~5  SaveName=ScopeData7
  mcnt : xps_library/software register  Tag=xps:sw_reg  io_dir=To Processor  arith_type=Unsigned  bitwidth=32  bin_pt=0  sample_period=1  gw_name=test_loopback_buf_loopback_mux_no_timeout_mcnt_user_data_in
  mcnt_verify : Scope  NumInputPorts=7
      settings: YMin=300~190.95~0~-5~-5~-5~-5  YMax=525~211.05~1~5~5~5~5  SaveName=ScopeData2
  posedge : casper_library/Misc/posedge  Tag=Rising Edge Detector
  posedge1 : casper_library/Misc/posedge  Tag=Rising Edge Detector
  rst_mcnt_regs : xps_library/software register  Tag=xps:sw_reg  io_dir=From Processor  arith_type=Unsigned  bitwidth=32  bin_pt=0  sample_period=1  gw_name=test_loopback_buf_loopback_mux_no_timeout_rst_mcnt_regs_user_data_out
  dout : Outport
  valid : Outport  Port=2
  eof : Outport  Port=3
  mcnt_out : Outport  Port=4
  ant_out : Outport  Port=5
  ip : Outport  Port=6
  loop_ack : Outport  Port=7
  gbe_ack : Outport  Port=8
  wires:
  Mux/1 -> dout/1
  Mux1/1 -> Convert/1
  Mux2/1 -> [eof_int], eof/1
  gbe_valid/1 -> Convert4/1
  loop_valid/1 -> Convert3/1
  Logical4/1 -> Mux2/2
  Logical1/1 -> Mux2/3
  Convert/1 -> valid/1
  gbe_mcnt/1 -> Mux4/2
  loop_mcnt/1 -> Mux5/2
  Slice2/1 -> Concat2/1
  Slice4/1 -> Concat2/2
  Concat2/1 -> mcnt/1
  Convert6/1 -> Mux/1
  Logical2/1 -> gbe_mcnt/3, Mux4/1
  Logical5/1 -> Mux5/1, loop_mcnt/3
  Slice/1 -> Convert1/1
  Constant1/1 -> rst_mcnt_regs/1
  rst_mcnt_regs/1 -> Slice5/1, Slice/1
  Slice5/1 -> posedge/1
  Convert1/1 -> Logical3/1
  [rst] -> loop_mcnt/2, gbe_mcnt/2
  [gbe_out_sel] -> Convert6/1
  [gbe_out_sel] -> Mux2/1
  [loop_rd_hdr] -> Logical5/1
  [gbe_rd_hdr] -> Logical2/1
  Counter/1 -> Slice6/1
  Slice6/1 -> posedge1/1
  [loop_out_sel] -> Counter/1
  Gateway Out12/1 -> loopback_mux_debug/3
  Gateway Out13/1 -> loopback_mux_debug/4
  Gateway Out14/1 -> loopback_mux_debug/5
  Gateway Out21/1 -> loopback_mux_debug/6
  Convert3/1 -> [loop_in_valid]
  Convert4/1 -> [gbe_in_valid]
  [loop_in_valid] -> Logical5/2
  [gbe_in_valid] -> Logical2/2
  [loop_in_valid] -> Logical4/1
  [gbe_in_valid] -> Logical1/1
  Relational1/1 -> [pkt_rdy]
  [pkt_rdy] -> Logical11/2
  loop_din/1 -> [loop_din]
  gbe_din/1 -> [gbe_din]
  posedge/1 -> Convert2/1
  Convert2/1 -> [rst]
  [loop_din] -> loop_mcnt/1, Mux5/3
  [gbe_din] -> gbe_mcnt/1, Mux4/3
  [loop_din] -> Mux/2
  [gbe_din] -> Mux/3
  [gbe_out_sel] -> gbe_ack/1
  [rst] -> Counter1/1
  Counter1/1 -> loop_timeouts/1
  [loop_out_sel] -> loop_ack/1
  [gbe_din] -> Gateway Out11/1
  [loop_din] -> Gateway Out10/1
  [loop_in_valid] -> Gateway Out12/1
  [gbe_in_valid] -> Gateway Out13/1
  [gbe_out_sel] -> Gateway Out21/1
  [pkt_rdy] -> Gateway Out14/1
  Gateway Out1/1 -> loopback_mux_debug/7
  [eof_int] -> Logical6/1
  [eof_int] -> Gateway Out1/1
  [loop_rd_hdr] -> Gateway Out2/1
  Gateway Out2/1 -> loopback_mux_debug/8
  Inverter3/1 -> [gbe_out_sel]
  in_sel/1 -> Convert7/1
  Logical6/1 -> in_sel/2
  Convert7/1 -> Inverter3/1, [loop_out_sel]
  [loop_in_valid] -> Logical11/1
  [loopback_rst] -> Logical6/2
  Logical3/1 -> [loopback_rst]
  Register2/1 -> Convert8/1
  Convert8/1 -> Inverter2/1
  Inverter2/1 -> [gbe_rd_hdr]
  [gbe_eof] -> Register2/2
  [loop_eof] -> Logical4/2
  loop_eof/1 -> Convert5/1
  gbe_eof/1 -> Convert10/1
  [gbe_eof] -> Logical1/2
  Register3/1 -> Convert9/1
  Convert9/1 -> Inverter4/1
  Inverter4/1 -> [loop_rd_hdr]
  [loop_eof] -> Register3/2
  Gateway Out3/1 -> loopback_mux_debug/9
  [gbe_rd_hdr] -> Gateway Out3/1
  Convert5/1 -> [loop_eof]
  Convert10/1 -> [gbe_eof]
  [gbe_out_sel] -> Convert11/1
  Convert11/1 -> Mux1/1
  loop_ip/1 -> [loop_ip]
  gbe_ip/1 -> [gbe_ip]
  Mux3/1 -> ip/1
  [loop_ip] -> Mux3/2
  [gbe_ip] -> Mux3/3
  [gbe_out_sel] -> Convert13/1
  Convert13/1 -> Mux3/1
  posedge1/1 -> Logical3/2, Counter1/2
  Logical/1 -> in_sel/1
  Logical11/1 -> Logical/2
  [loopback_rst] -> Logical/1
  Logical8/1 -> Register2/1, Register2/3
  [gbe_in_valid] -> Logical8/1
  [gbe_out_sel] -> Logical8/2
  Logical7/1 -> Register3/1, Register3/3
  [loop_in_valid] -> Logical7/1
  [loop_out_sel] -> Logical7/2
  [loop_mcnt] -> Slice2/1
  [gbe_mcnt] -> Slice4/1
  Gateway Out10/1 -> loopback_mux_debug/1
  Gateway Out11/1 -> loopback_mux_debug/2
  Gateway Out4/1 -> loopback_mux_debug/10
  Gateway Out5/1 -> loopback_mux_debug/11
  [loop_mcnt] -> Gateway Out4/1
  [gbe_mcnt] -> Gateway Out5/1
  Gateway Out24/1 -> mcnt_verify/3
  Gateway Out22/1 -> mcnt_verify/1
  Gateway Out23/1 -> mcnt_verify/2
  Gateway Out25/1 -> mcnt_verify/4
  Gateway Out18/1 -> mcnt_verify/5
  Gateway Out19/1 -> mcnt_verify/6
  Gateway Out20/1 -> mcnt_verify/7
  [gbe_out_sel] -> Gateway Out20/1
  [gbe_in_valid] -> Gateway Out19/1
  [loop_in_valid] -> Gateway Out18/1
  [eof_int] -> Gateway Out25/1
  [loop_mcnt] -> Gateway Out22/1
  [gbe_mcnt] -> Gateway Out23/1
  [pkt_rdy] -> Gateway Out24/1
  Mux4/1 -> Slice8/1, [gbe_hdr]
  Mux5/1 -> Slice7/1, [loop_hdr]
  [gbe_in_valid] -> Inverter1/1
  [loop_in_valid] -> Inverter5/1
  Logical9/1 -> Logical6/3
  Inverter1/1 -> Logical9/1
  Inverter5/1 -> Logical9/2
  [loop_rd_hdr] -> Logical9/3
  [gbe_rd_hdr] -> Logical9/4
  Slice7/1 -> Relational1/1, [loop_mcnt]
  Slice8/1 -> Relational1/2, [gbe_mcnt]
  Slice1/1 -> mcnt_out/1
  Slice3/1 -> ant_out/1
  Convert12/1 -> Mux6/1
  [gbe_out_sel] -> Convert12/1
  [loop_hdr] -> Mux6/2
  [gbe_hdr] -> Mux6/3
  Mux6/1 -> Slice1/1, Slice3/1
  Inverter6/1 -> Logical10/1
  Logical10/1 -> Mux1/2
  [loop_in_valid] -> Logical10/2
  [loop_rd_hdr] -> Inverter6/1
  [gbe_rd_hdr] -> Inverter7/1
  [gbe_in_valid] -> Logical12/2
  Logical12/1 -> Mux1/3
  Inverter7/1 -> Logical12/1
